simulink model "LMI"  (R2026b)
settings: Solver=ode4  StopTime=10  FixedStep=1e-4
values from neighbouring files (symbols this model uses):
  K = f*p    [Ganancias.m]
  K2 = f*p    [Ganancias.m]
settings Model: Creator=Yahoff  LastModifiedBy=Yahoff

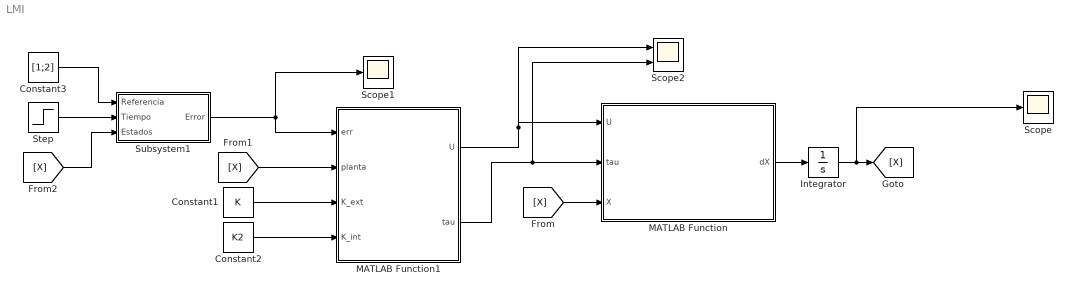
== system LMI ==
  Constant1 : Constant  Value=K
  Constant2 : Constant  Value=K2
  Constant3 : Constant  Value=[1;2]
  Integrator : Integrator  InitialCondition=[0;0;0;0;0;0]
  MATLAB Function : MATLAB Function  TreatAsAtomicUnit=on
  MATLAB Function1 : MATLAB Function  TreatAsAtomicUnit=on
  Scope : Scope
      settings: ActiveDisplayYMinimum=-11.56695387739583  ActiveDisplayYMaximum=24.402802551431083
  Scope1 : Scope
      settings: ActiveDisplayYMinimum=-12610.15580763148  ActiveDisplayYMaximum=4381.1497291038568
  Scope2 : Scope  NumInputPorts=2
      settings: ActiveDisplayYMinimum=-41.769638728880224  ActiveDisplayYMaximum=356.28339104262261  DataLoggingVariableName=ScopeData2
  Step : Step  SampleTime=0
  Subsystem1 : Subsystem
  wires:
  MATLAB Function/1(dX) -> Integrator/1
  Integrator/1 -> Scope/1, [X]
  [X] -> MATLAB Function/3(X)
  [X] -> MATLAB Function1/2(planta)
  MATLAB Function1/1(U) -> Scope2/1, MATLAB Function/1(U)
  MATLAB Function1/2(tau) -> Scope2/2, MATLAB Function/2(tau)
  [X] -> Subsystem1/3(Estados)
  Constant3/1 -> Subsystem1/1(Referencia)
  Step/1 -> Subsystem1/2(Tiempo)
  Subsystem1/1(Error) -> Scope1/1, MATLAB Function1/1(err)
  Constant2/1 -> MATLAB Function1/4(K_int)
  Constant1/1 -> MATLAB Function1/3(K_ext)

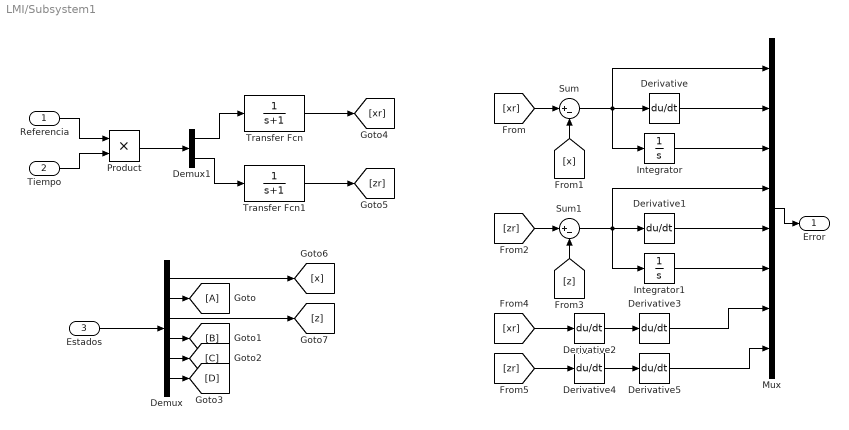
== system LMI/Subsystem1 ==
  Referencia : Inport
  Tiempo : Inport  Port=2
  Estados : Inport  Port=3
  Demux : Demux  Outputs=6
  Demux1 : Demux  Outputs=2
  Derivative{,1..5} (6 alike) : Derivative
  Goto : Goto
  Integrator : Integrator
  Integrator1 : Integrator
  Mux : Mux  Inputs=8
  Product : Product
  Sum : Sum  Inputs=|+-
  Sum1 : Sum  Inputs=|+-
  Transfer Fcn : TransferFcn  Denominator=[1 1]
  Transfer Fcn1 : TransferFcn  Denominator=[1 1]
  Error : Outport
  wires:
  Demux/3 -> [z]
  Demux/1 -> [x]
  Demux/5 -> [C]
  Demux/6 -> [D]
  Estados/1 -> Demux/1
  Demux/2 -> Goto/1
  Demux/4 -> [B]
  Referencia/1 -> Product/1
  Tiempo/1 -> Product/2
  Product/1 -> Demux1/1
  Demux1/2 -> Transfer Fcn1/1
  Demux1/1 -> Transfer Fcn/1
  Transfer Fcn/1 -> [xr]
  Transfer Fcn1/1 -> [zr]
  [xr] -> Sum/1
  [x] -> Sum/2
  [zr] -> Sum1/1
  [z] -> Sum1/2
  Sum/1 -> Derivative/1, Integrator/1, Mux/1
  Sum1/1 -> Derivative1/1, Integrator1/1, Mux/4
  Integrator/1 -> Mux/3
  Integrator1/1 -> Mux/6
  Mux/1 -> Error/1
  Derivative/1 -> Mux/2
  Derivative1/1 -> Mux/5
  [xr] -> Derivative2/1
  Derivative2/1 -> Derivative3/1
  Derivative4/1 -> Derivative5/1
  [zr] -> Derivative4/1
  Derivative3/1 -> Mux/7
  Derivative5/1 -> Mux/8

== matlab function LMI/MATLAB Function1 ==
  data: err input; U output; planta input; tau output; K_ext input; K_int input
function [U, tau] = control(err, planta, K_ext, K_int)

m = 1; g = 9.81;

% Entradas
ex    = err(1);
dex   = err(2);
Iex   = err(3);
ez    = err(4);
dez   = err(5);
Iez   = err(6);
xrdd  = err(7);
zrdd  = err(8);

x     = planta(1);
xdot  = planta(2);
z     = planta(3);
zdot  = planta(4);
th    = planta(5);
thdot = planta(6);

% Lazo externo con acción integral
vx = xrdd - K_ext(1)*ex - K_ext(2)*dex - K_ext(3)*Iex;
vz = zrdd - K_ext(1)*ez - K_ext(2)*dez - K_ext(3)*Iez;

% Conversión
U   = m*sqrt(vx^2 + (vz+g)^2);
thd = atan2(-vx, vz+g);

% Lazo interno
eth  = th - thd;
deth = thdot;
tau  = -K_int(1)*eth - K_int(2)*deth;
end

== matlab function LMI/MATLAB Function ==
  data: U input; dX output; tau input; X input
function dX = planta(U, tau, X)

    m = 1; J = 1; g = 9.81;
    kth = 30; kom = 12;

    x     = X(1);
    xdot  = X(2);
    z     = X(3);
    zdot  = X(4);
    th    = X(5);
    thdot = X(6);

    xdd  = -(U/m)*sin(th);
    zdd  =  (U/m)*cos(th) - g;
    thdd =  tau/J;

    dX = [xdot; xdd; zdot; zdd; thdot; thdd];
